simulink model "MDCC"  (R2021b)
settings: Solver=FixedStepDiscrete  StartTime=0.0  StopTime=10.0  FixedStep=0.0001  RelTol=1e-3
model workspace (MATLAB code in the model file):
  | cmdLim = Simulink.Parameter;
  | cmdLim.Value = 15;
  | cmdLim.Description = 'Limit for controlling the maximum surface command angle.';
  | cmdLim.Min = 0;
  | cmdLim.Max = 90;
  | cmdLim.DocUnits = 'deg';
  | 
  | dispGain = Simulink.Parameter;
  | dispGain.Value = 0.75;
  | dispGain.Description = 'Gain applied to the displacement error.';
  | dispGain.Min = 0;
  | dispGain.Max = [];
  | dispGain.DocUnits = 'deg/sec/deg';
  | 
  | dispLim = Simulink.Parameter;
  | dispLim.Value = 30;
  | dispLim.Description = 'Limit for controlling the maximum commanded angle.';
  | dispLim.Min = 0;
  | dispLim.Max = 180;
  | dispLim.DocUnits = 'deg';
  | 
  | intGain = Simulink.Parameter;
  | intGain.Value = 0.5;
  | intGain.Description = 'Gain applied to the integral error.';
  | intGain.Min = 0;
  | intGain.Max = [];
  | intGain.DocUnits = 'deg/sec/deg/sec';
  | 
  | intLim = Simulink.Parameter;
  | intLim.Value = 5;
  | intLim.Description = 'Limit for controlling the maximum commanded angle.';
  | intLim.Min = 0;
  | intLim.Max = 90;
  | intLim.DocUnits = 'deg';
  | 
  | rateGain = Simulink.Parameter;
  | rateGain.Value = 2;
  | rateGain.Description = 'Gain applied to the rate error.';
  | rateGain.Min = 0;
  | rateGain.Max = [];
  | rateGain.DocUnits = 'deg/deg/sec';
  | 
  | rateLim = Simulink.Parameter;
  | rateLim.Value = 6;
  | rateLim.Description = 'Limit for controlling the maximum commanded angle.';
  | rateLim.Min = 0;
  | rateLim.Max = 180;
  | rateLim.DocUnits = 'deg/sec';
  | 
  | hdgGain = Simulink.Parameter;
  | hdgGain.Value = 0.015;
values from neighbouring files (symbols this model uses):
  KfDeadCompen_SetDeltaTime_us = myPackage.Parameter    [DeadCompen.m]
  Ts = 5E-6    (= 5e-06)    [iPMSM_data.m]
  VbDeadComp_SwtUseIsttrDes_flg = myPackage.Parameter    [DeadCompen.m]
  VfDeadCompen_ISttrDdeThdSwt_A = myPackage.Parameter    [DeadCompen.m]
  VfDeadCompen_ISttrIgbtThdSwt_A = myPackage.Parameter    [DeadCompen.m]
  VfDeadCompen_rDdeISttrHi_R = myPackage.Parameter    [DeadCompen.m]
  VfDeadCompen_rDdeISttrLo_R = myPackage.Parameter    [DeadCompen.m]
  VfDeadCompen_rIgbtISttrHi_R = myPackage.Parameter    [DeadCompen.m]
  VfDeadCompen_rIgbtISttrLo_R = myPackage.Parameter    [DeadCompen.m]
  VfDeadCompen_uDdeISttrHi_V = myPackage.Parameter    [DeadCompen.m]
  VfDeadCompen_uDdeISttrLo_V = myPackage.Parameter    [DeadCompen.m]
  VfDeadCompen_uIgbtISttrHi_V = myPackage.Parameter    [DeadCompen.m]
  VfDeadCompen_uIgbtISttrLo_V = myPackage.Parameter    [DeadCompen.m]
undefined symbols (not defined in the file or in its folder): CosTable12bit_Y, GLBCal_GLBCal_Kf_DCLinkOverVolErrThd_V, GLBCal_GLBCal_Kf_DCLinkUnderVolErrThd_V, GLBCal_GLBCal_Kf_EquiLd_NULL, GLBCal_GLBCal_Kf_EquiLq_NULL, GLBCal_GLBCal_Kf_MotorRatedSpeed_rpm, GLBCal_GLBCal_Kf_MotorSpeedHysteresis_Coef, GLBCal_Ke_MotorPolePairsNum_NULL, IoHwAbOpArg_PwmDutyCyclePhU_NULL, IoHwAbOpArg_PwmDutyCyclePhV_NULL, IoHwAbOpArg_PwmDutyCyclePhW_NULL, IoHwAbOpArg_PwmOutputEn, KbMDCC_DeadTimeCompEn_flg, KbMDCC_MCF_flgHarmInIsdqTab11ZR_flg, KbMDCC_MCF_flgHarmInIsdqTab13ZR_flg, KbMDCC_MCF_flgHarmInIsdqTab5ZR_flg, KbMDCC_MCF_flgHarmInIsdqTab7ZR_flg, KbMDCC_MCF_flgHarmInject_flg, KbMDCC_SetEAngleEn_flg, KbMDCC_UdUqFwOmit_flg, KfDeadCompen_CpPeriodTimesT_NULL, KfMDCC_ActiveDischargeIdCurVal_A, KfMDCC_ActiveDischargeIqCurVal_A, KfMDCC_DCLinkVolRate_coef, KfMDCC_DebugEAngleInit_rad, KfMDCC_DebugUalphaVolCmd_V, KfMDCC_DebugUbetaVolCmd_V, KfMDCC_DebugUdCmd_V, KfMDCC_DebugUqCmd_V, KfMDCC_DebugUsCmd_V, KfMDCC_DebugUsRate_V, KfMDCC_IMCResp_NULL, KfMDCC_IMCStab_NULL, KfMDCC_InvParkCpPeriodTimesT_NULL, KfMDCC_MCF_CircAge_NULL, KfMDCC_MCF_flgUse11Harm_flg, KfMDCC_MCF_flgUse13Harm_flg, KfMDCC_MCF_flgUse5Harm_flg, KfMDCC_MCF_flgUse7Harm_flg, KfMDCC_MCF_Harm1113FLParamSpeedThrd_rads, KfMDCC_MCF_Harm57FLParamSpeedThrd_rads, KfMDCC_MCF_HarmcofFltN_NULL, KfMDCC_MCF_HarmCpnAg_NULL, KfMDCC_MCF_HarmfLParaHigh_coef, KfMDCC_MCF_HarmfLParaLow_coef, KfMDCC_MCF_HarmIn1113ZRY_Trq_Nm, KfMDCC_MCF_HarmIn11_SpdLimHigh_rads, KfMDCC_MCF_HarmIn11_SpdLimLow_rads, KfMDCC_MCF_HarmIn11ZRY_Isd_A, KfMDCC_MCF_HarmIn11ZRY_Isq_A, KfMDCC_MCF_HarmIn13_SpdLimHigh_rads, KfMDCC_MCF_HarmIn13_SpdLimLow_rads, KfMDCC_MCF_HarmIn13ZRY_Isd_A, KfMDCC_MCF_HarmIn13ZRY_Isq_A, KfMDCC_MCF_HarmIn57ZRY_Trq_Nm, KfMDCC_MCF_HarmIn5_SpdLimHigh_rads, KfMDCC_MCF_HarmIn5_SpdLimLow_rads, KfMDCC_MCF_HarmIn5ZRY_Isd_A, KfMDCC_MCF_HarmIn5ZRY_Isq_A, KfMDCC_MCF_HarmIn7_SpdLimHigh_rads ... (+47)
libraries: simulink x40, PMSM_Library x3, mcbcontrolslib x1
(part 5 of 8)

== system MDCC/DoCurCtr_sys/MDCC/UdUqCalc_Sys/MDCC_MCF_Sys/Enabled Subsystem/Harmonic_Injection_11/Subsystem ==
  MCF_Harm_isdDes11 : Inport
  MCF_Harm_isqDes11 : Inport  Port=2
  MCF_Harm_isdAct11 : Inport  Port=3
  MCF_Harm_isqAct11 : Inport  Port=4
  MCF_Sin11Ag : Inport  Port=5
  MCF_Cos11Ag : Inport  Port=6
  Rdc_absnWoFlt_rads : Inport  Port=7
  MCF_flgHarm11PIRest : Inport  Port=8
  ZeroEnable : EnablePort
  Harm_11Step_KpKi : Subsystem
  RevPark : Subsystem
  MCF_uAlpha_Harm11 : Outport  VectorParamsAs1DForOutWhenUnconnected=off
  MCF_uBeta_Harm11 : Outport  Port=2  VectorParamsAs1DForOutWhenUnconnected=off
  wires:
  MCF_Harm_isqDes11/1 -> Harm_11Step_KpKi/2(MCF_Harm_isqDes11)
  MCF_Harm_isqAct11/1 -> Harm_11Step_KpKi/4(MCF_Harm_isqAct11)
  RevPark/2(MCF_uBeta_Harm11) -> MCF_uBeta_Harm11/1
  MCF_Harm_isdAct11/1 -> Harm_11Step_KpKi/3(MCF_Harm_isdAct11)
  RevPark/1(MCF_uAlpha_Harm11) -> MCF_uAlpha_Harm11/1
  MCF_Harm_isdDes11/1 -> Harm_11Step_KpKi/1(MCF_Harm_isdDes11)
  MCF_flgHarm11PIRest/1 -> Harm_11Step_KpKi/6(MCF_flgHarm11PIRest)
  Rdc_absnWoFlt_rads/1 -> Harm_11Step_KpKi/5(Rdc_absnWoFlt_rads)
  Harm_11Step_KpKi/1(MCF_Harm_ud11PI) -> RevPark/1(MCF_Harm_ud11PI)
  Harm_11Step_KpKi/2(MCF_Harm_uq11PI) -> RevPark/2(MCF_Harm_uq11PI)
  MCF_Sin11Ag/1 -> RevPark/3(MCF_Sin11Ag)
  MCF_Cos11Ag/1 -> RevPark/4(MCF_Cos11Ag)

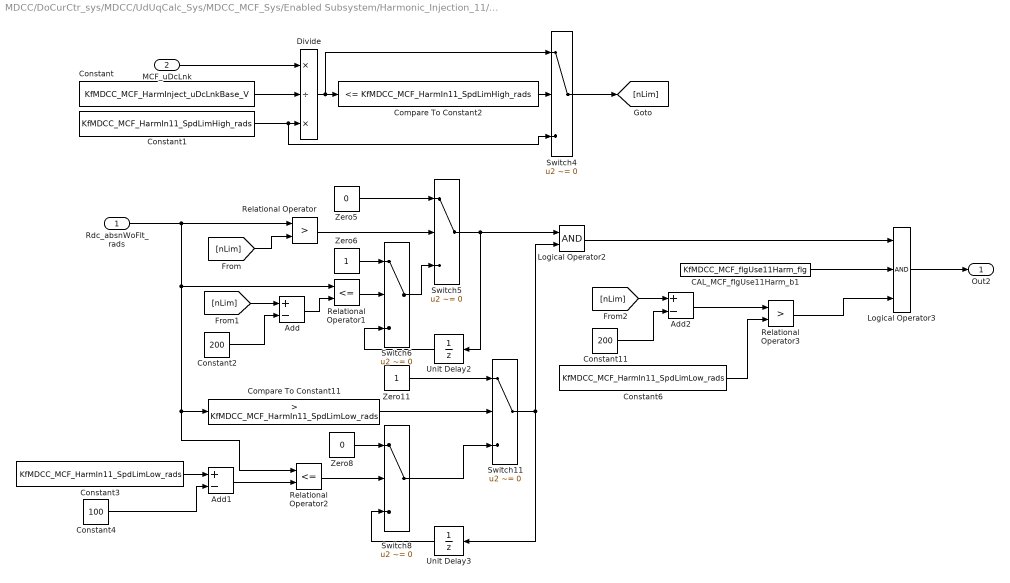
== system MDCC/DoCurCtr_sys/MDCC/UdUqCalc_Sys/MDCC_MCF_Sys/Enabled Subsystem/Harmonic_Injection_11/Subsystem1 ==
  Rdc_absnWoFlt_rads : Inport
  MCF_uDcLnk : Inport  Port=2
  Add : Sum  Inputs=+-
  Add1 : Sum  Inputs=+-
  Add2 : Sum  Inputs=+-
  CAL_MCF_flgUse11Harm_b1 : Constant  Value=KfMDCC_MCF_flgUse11Harm_flg
  Compare To Constant11 : simulink/Logic and Bit Operations/Compare To Constant  relop=>  const=KfMDCC_MCF_HarmIn11_SpdLimLow_rads  OutDataTypeStr=boolean
  Compare To Constant2 : simulink/Logic and Bit Operations/Compare To Constant  relop=<=  const=KfMDCC_MCF_HarmIn11_SpdLimHigh_rads  OutDataTypeStr=boolean
  Constant : Constant  Value=KfMDCC_MCF_HarmInject_uDcLnkBase_V
  Constant1 : Constant  Value=KfMDCC_MCF_HarmIn11_SpdLimHigh_rads
  Constant11 : Constant  Value=200  OutDataTypeStr=single
  Constant2 : Constant  Value=200  OutDataTypeStr=single
  Constant3 : Constant  Value=KfMDCC_MCF_HarmIn11_SpdLimLow_rads
  Constant4 : Constant  Value=100  OutDataTypeStr=single
  Constant6 : Constant  Value=KfMDCC_MCF_HarmIn11_SpdLimLow_rads
  Divide : Product  Inputs=*/*
  Logical Operator2 : Logic  AllPortsSameDT=off  OutDataTypeStr=boolean
  Logical Operator3 : Logic  Inputs=3  AllPortsSameDT=off  OutDataTypeStr=boolean
  Relational Operator : RelationalOperator  Operator=>  OutDataTypeStr=boolean  RndMeth=Simplest
  Relational Operator1 : RelationalOperator  Operator=<=  OutDataTypeStr=boolean  RndMeth=Simplest
  Relational Operator2 : RelationalOperator  Operator=<=  OutDataTypeStr=boolean  RndMeth=Simplest
  Relational Operator3 : RelationalOperator  Operator=>  OutDataTypeStr=boolean  RndMeth=Simplest
  Switch{4..6,8,11} (5 alike) : Switch  Criteria=u2 ~= 0
  Unit Delay2 : UnitDelay  SampleTime=-1  HasFrameUpgradeWarning=on
  Unit Delay3 : UnitDelay  SampleTime=-1  HasFrameUpgradeWarning=on
  Zero11 : Constant  OutDataTypeStr=boolean
  Zero5 : Constant  Value=0  OutDataTypeStr=boolean
  Zero6 : Constant  OutDataTypeStr=boolean
  Zero8 : Constant  Value=0  OutDataTypeStr=boolean
  Out2 : Outport
  wires:
  Constant/1 -> Divide/2
  MCF_uDcLnk/1 -> Divide/1
  Constant1/1 -> Switch4/3, Divide/3
  Divide/1 -> Switch4/1, Compare To Constant2/1
  Compare To Constant2/1 -> Switch4/2
  Switch4/1 -> [nLim]
  CAL_MCF_flgUse11Harm_b1/1 -> Logical Operator3/2
  Relational Operator2/1 -> Switch8/2
  Relational Operator1/1 -> Switch6/2
  Switch8/1 -> Switch11/3
  Compare To Constant11/1 -> Switch11/2
  Unit Delay3/1 -> Switch8/3
  Switch11/1 -> Unit Delay3/1, Logical Operator2/2
  Relational Operator/1 -> Switch5/2
  Switch5/1 -> Logical Operator2/1, Unit Delay2/1
  Zero6/1 -> Switch6/1
  Logical Operator3/1 -> Out2/1
  Switch6/1 -> Switch5/3
  Zero11/1 -> Switch11/1
  Unit Delay2/1 -> Switch6/3
  Zero8/1 -> Switch8/1
  Rdc_absnWoFlt_rads/1 -> Relational Operator/1, Relational Operator2/1, Compare To Constant11/1, Relational Operator1/1
  Logical Operator2/1 -> Logical Operator3/1
  Zero5/1 -> Switch5/1
  [nLim] -> Relational Operator/2
  [nLim] -> Add/1
  Add/1 -> Relational Operator1/2
  Constant2/1 -> Add/2
  Constant3/1 -> Add1/1
  Constant4/1 -> Add1/2
  Add1/1 -> Relational Operator2/2
  [nLim] -> Add2/1
  Constant11/1 -> Add2/2
  Add2/1 -> Relational Operator3/1
  Constant6/1 -> Relational Operator3/2
  Relational Operator3/1 -> Logical Operator3/3

== system MDCC/DoCurCtr_sys/MDCC/UdUqCalc_Sys/MDCC_MCF_Sys/Enabled Subsystem/Harmonic_Injection_11/Subsystem2 ==
  TDC_TrqDes : Inport
  flgHarmUse : Inport  Port=2
  Add : Sum  Inputs=+-
  Add1 : Sum  Inputs=-+
  Add2 : Sum  Inputs=-+
  Add3 : Sum
  Compare To Constant : simulink/Logic and Bit Operations/Compare To Constant  relop=>=  const=KfMDCC_MCF_TrqFltCof_NULL  OutDataTypeStr=boolean
  Compare To Constant1 : simulink/Logic and Bit Operations/Compare To Constant  relop=>=  const=KfMDCC_MCF_TrqFltCof_NULL  OutDataTypeStr=boolean
  Constant : Constant  Value=KfMDCC_MCF_TrqFlt_coef  OutDataTypeStr=single
  Switch : Switch  Criteria=u2 > Threshold
  Switch1 : Switch  Criteria=u2 > Threshold
  Switch2 : Switch  Criteria=u2 ~= 0
  Unit Delay : UnitDelay  SampleTime=-1  HasFrameUpgradeWarning=on
  Unit Delay1 : UnitDelay  SampleTime=-1  HasFrameUpgradeWarning=on
  Zero : Constant  Value=0  OutDataTypeStr=single
  TDC_TrqDesFlt : Outport
  wires:
  Add/1 -> Compare To Constant/1
  Compare To Constant/1 -> Switch/2
  Add1/1 -> Switch/1
  Switch/1 -> Switch2/1
  TDC_TrqDes/1 -> Switch1/3, Add2/2, Add/2
  Add2/1 -> Compare To Constant1/1
  Constant/1 -> Add1/1, Add3/1
  Add3/1 -> Switch1/1
  Compare To Constant1/1 -> Switch1/2
  Switch1/1 -> Switch/3
  Unit Delay/1 -> Add/1, Add1/2, Add2/1, Add3/2
  flgHarmUse/1 -> Unit Delay1/1
  Unit Delay1/1 -> Switch2/2
  Zero/1 -> Switch2/3
  Switch2/1 -> Unit Delay/1, TDC_TrqDesFlt/1

== system MDCC/DoCurCtr_sys/MDCC/UdUqCalc_Sys/MDCC_MCF_Sys/Enabled Subsystem/Harmonic_Injection_13/Set_13_steps_current_isdqdes ==
  TDC_TrqDesFlt : Inport
  1-D Lookup Table : Lookup_n-D  NumberOfTableDimensions=1  BreakpointsForDimension1=KfMDCC_MCF_HarmIn1113ZRY_Trq_Nm  Table=KfMDCC_MCF_HarmIn13ZRY_Isd_A  InternalRulePriority=Speed  RndMeth=Simplest  InputSameDT=on
  1-D Lookup Table1 : Lookup_n-D  NumberOfTableDimensions=1  BreakpointsForDimension1=KfMDCC_MCF_HarmIn1113ZRY_Trq_Nm  Table=KfMDCC_MCF_HarmIn13ZRY_Isq_A  InternalRulePriority=Speed  RndMeth=Simplest  InputSameDT=on
  Bus Creator1 : BusCreator  Inputs=2
  Bus Creator2 : BusCreator  Inputs=2
  Bus Selector1 : BusSelector  OutputSignals=MCF_IsdDes13Harm_A,MCF_IsqDes13Harm_A
  CAL_MCF_IsDes13Harm_f32 : Constant  Value=KfMDCC_MCF_IsDes13Harm_A
  CAL_MCF_IsThetaDes13Harm_f32 : Constant  Value=KfMDCC_MCF_IsThetaDes13Harm_NULL
  CAL_MCF_flgHarmInIsdqTab13ZR_b : Constant  Value=KbMDCC_MCF_flgHarmInIsdqTab13ZR_flg
  LookUpEAngleCosSin2 : Subsystem  TreatAsAtomicUnit=on  RTWFcnName=MCF_MDCC_LookUpEAngleCosSin  RTWFileName=MDCC
      settings: RTWFcnNameOpts=User specified
  Product13 : Product  OutDataTypeStr=uint16
  Product2 : Product
  Product5 : Product
  Signal Copy : SignalConversion  OverrideOpt=off
  Signal Copy1 : SignalConversion  OverrideOpt=off
  Sine_and_cosine_table1 : Constant  Value=13.31313  OutDataTypeStr=single
  Switch1 : Switch  Criteria=u2 ~= 0
  VfMDCC_MCF_IsdDes13Harm_A : Outport  VectorParamsAs1DForOutWhenUnconnected=off
  VfMDCC_MCF_IsqDes13Harm_A : Outport  Port=2  VectorParamsAs1DForOutWhenUnconnected=off
  wires:
  Signal Copy1/1 -> VfMDCC_MCF_IsqDes13Harm_A/1  "VfMDCC_MCF_IsqDes13Harm_A"
  Signal Copy/1 -> VfMDCC_MCF_IsdDes13Harm_A/1  "VfMDCC_MCF_IsdDes13Harm_A"
  Bus Selector1/2 -> Signal Copy1/1  "<MCF_IsqDes13Harm_A>"
  Bus Selector1/1 -> Signal Copy/1  "<MCF_IsdDes13Harm_A>"
  Switch1/1 -> Bus Selector1/1
  CAL_MCF_flgHarmInIsdqTab13ZR_b/1 -> Switch1/2
  1-D Lookup Table1/1 -> Bus Creator2/2  "MCF_IsqDes13Harm_A"
  Bus Creator2/1 -> Switch1/1
  1-D Lookup Table/1 -> Bus Creator2/1  "MCF_IsdDes13Harm_A"
  TDC_TrqDesFlt/1 -> 1-D Lookup Table/1, 1-D Lookup Table1/1
  CAL_MCF_IsDes13Harm_f32/1 -> Product5/1, Product2/1
  Sine_and_cosine_table1/1 -> Product13/2
  LookUpEAngleCosSin2/2(VfMDCC_EAngleSin_NULL) -> Product5/2
  Product2/1 -> Bus Creator1/1  "MCF_IsdDes13Harm_A"
  Bus Creator1/1 -> Switch1/3
  Product13/1 -> LookUpEAngleCosSin2/1(VuMDCC_MotorPositionCnt_NULL)
  CAL_MCF_IsThetaDes13Harm_f32/1 -> Product13/1
  Product5/1 -> Bus Creator1/2  "MCF_IsqDes13Harm_A"
  LookUpEAngleCosSin2/1(VfMDCC_EAngleCos_NULL) -> Product2/2

== system MDCC/DoCurCtr_sys/MDCC/UdUqCalc_Sys/MDCC_MCF_Sys/Enabled Subsystem/Harmonic_Injection_13/Subsystem ==
  MCF_Harm_isdDes13 : Inport
  MCF_Harm_isqDes13 : Inport  Port=2
  MCF_Harm_isdAct13 : Inport  Port=3
  MCF_Harm_isqAct13 : Inport  Port=4
  MCF_Sin13Ag : Inport  Port=5
  MCF_Cos13Ag : Inport  Port=6
  Rdc_absnWoFlt_rads : Inport  Port=7
  MCF_flgHarm13PIRest : Inport  Port=8
  ZeroEnable : EnablePort
  Harm_13Step_KpKi : Subsystem
  RevPark : Subsystem
  MCF_uAlpha_Harm13 : Outport  VectorParamsAs1DForOutWhenUnconnected=off
  MCF_uBeta_Harm13 : Outport  Port=2  VectorParamsAs1DForOutWhenUnconnected=off
  wires:
  MCF_Harm_isqDes13/1 -> Harm_13Step_KpKi/2(MCF_Harm_isqDes13)
  MCF_Harm_isqAct13/1 -> Harm_13Step_KpKi/4(MCF_Harm_isqAct13)
  RevPark/2(MCF_uBeta_Harm13) -> MCF_uBeta_Harm13/1
  MCF_Harm_isdAct13/1 -> Harm_13Step_KpKi/3(MCF_Harm_isdAct13)
  RevPark/1(MCF_uAlpha_Harm13) -> MCF_uAlpha_Harm13/1
  MCF_Harm_isdDes13/1 -> Harm_13Step_KpKi/1(MCF_Harm_isdDes13)
  MCF_flgHarm13PIRest/1 -> Harm_13Step_KpKi/6(MCF_flgHarm13PIRest)
  Rdc_absnWoFlt_rads/1 -> Harm_13Step_KpKi/5(Rdc_absnWoFlt_rads)
  Harm_13Step_KpKi/1(MCF_Harm_ud13PI) -> RevPark/1(MCF_Harm_ud13PI)
  Harm_13Step_KpKi/2(MCF_Harm_uq13PI) -> RevPark/2(MCF_Harm_uq13PI)
  MCF_Sin13Ag/1 -> RevPark/3(MCF_Sin13Ag)
  MCF_Cos13Ag/1 -> RevPark/4(MCF_Cos13Ag)

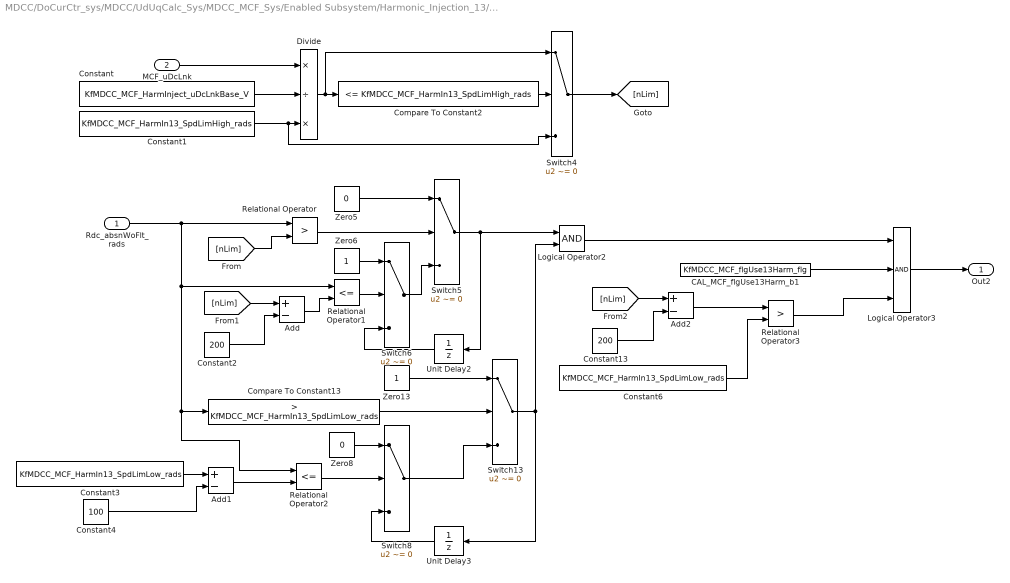
== system MDCC/DoCurCtr_sys/MDCC/UdUqCalc_Sys/MDCC_MCF_Sys/Enabled Subsystem/Harmonic_Injection_13/Subsystem1 ==
  Rdc_absnWoFlt_rads : Inport
  MCF_uDcLnk : Inport  Port=2
  Add : Sum  Inputs=+-
  Add1 : Sum  Inputs=+-
  Add2 : Sum  Inputs=+-
  CAL_MCF_flgUse13Harm_b1 : Constant  Value=KfMDCC_MCF_flgUse13Harm_flg
  Compare To Constant13 : simulink/Logic and Bit Operations/Compare To Constant  relop=>  const=KfMDCC_MCF_HarmIn13_SpdLimLow_rads  OutDataTypeStr=boolean
  Compare To Constant2 : simulink/Logic and Bit Operations/Compare To Constant  relop=<=  const=KfMDCC_MCF_HarmIn13_SpdLimHigh_rads  OutDataTypeStr=boolean
  Constant : Constant  Value=KfMDCC_MCF_HarmInject_uDcLnkBase_V
  Constant1 : Constant  Value=KfMDCC_MCF_HarmIn13_SpdLimHigh_rads
  Constant13 : Constant  Value=200  OutDataTypeStr=single
  Constant2 : Constant  Value=200  OutDataTypeStr=single
  Constant3 : Constant  Value=KfMDCC_MCF_HarmIn13_SpdLimLow_rads
  Constant4 : Constant  Value=100  OutDataTypeStr=single
  Constant6 : Constant  Value=KfMDCC_MCF_HarmIn13_SpdLimLow_rads
  Divide : Product  Inputs=*/*
  Logical Operator2 : Logic  AllPortsSameDT=off  OutDataTypeStr=boolean
  Logical Operator3 : Logic  Inputs=3  AllPortsSameDT=off  OutDataTypeStr=boolean
  Relational Operator : RelationalOperator  Operator=>  OutDataTypeStr=boolean  RndMeth=Simplest
  Relational Operator1 : RelationalOperator  Operator=<=  OutDataTypeStr=boolean  RndMeth=Simplest
  Relational Operator2 : RelationalOperator  Operator=<=  OutDataTypeStr=boolean  RndMeth=Simplest
  Relational Operator3 : RelationalOperator  Operator=>  OutDataTypeStr=boolean  RndMeth=Simplest
  Switch{4..6,8,13} (5 alike) : Switch  Criteria=u2 ~= 0
  Unit Delay2 : UnitDelay  SampleTime=-1  HasFrameUpgradeWarning=on
  Unit Delay3 : UnitDelay  SampleTime=-1  HasFrameUpgradeWarning=on
  Zero13 : Constant  OutDataTypeStr=boolean
  Zero5 : Constant  Value=0  OutDataTypeStr=boolean
  Zero6 : Constant  OutDataTypeStr=boolean
  Zero8 : Constant  Value=0  OutDataTypeStr=boolean
  Out2 : Outport
  wires:
  Constant/1 -> Divide/2
  MCF_uDcLnk/1 -> Divide/1
  Constant1/1 -> Switch4/3, Divide/3
  Divide/1 -> Switch4/1, Compare To Constant2/1
  Compare To Constant2/1 -> Switch4/2
  Switch4/1 -> [nLim]
  CAL_MCF_flgUse13Harm_b1/1 -> Logical Operator3/2
  Relational Operator2/1 -> Switch8/2
  Relational Operator1/1 -> Switch6/2
  Switch8/1 -> Switch13/3
  Compare To Constant13/1 -> Switch13/2
  Unit Delay3/1 -> Switch8/3
  Switch13/1 -> Unit Delay3/1, Logical Operator2/2
  Relational Operator/1 -> Switch5/2
  Switch5/1 -> Logical Operator2/1, Unit Delay2/1
  Zero6/1 -> Switch6/1
  Logical Operator3/1 -> Out2/1
  Switch6/1 -> Switch5/3
  Zero13/1 -> Switch13/1
  Unit Delay2/1 -> Switch6/3
  Zero8/1 -> Switch8/1
  Rdc_absnWoFlt_rads/1 -> Relational Operator/1, Relational Operator2/1, Compare To Constant13/1, Relational Operator1/1
  Logical Operator2/1 -> Logical Operator3/1
  Zero5/1 -> Switch5/1
  [nLim] -> Relational Operator/2
  [nLim] -> Add/1
  Add/1 -> Relational Operator1/2
  Constant2/1 -> Add/2
  Constant3/1 -> Add1/1
  Constant4/1 -> Add1/2
  Add1/1 -> Relational Operator2/2
  [nLim] -> Add2/1
  Constant13/1 -> Add2/2
  Add2/1 -> Relational Operator3/1
  Constant6/1 -> Relational Operator3/2
  Relational Operator3/1 -> Logical Operator3/3

== system MDCC/DoCurCtr_sys/MDCC/UdUqCalc_Sys/MDCC_MCF_Sys/Enabled Subsystem/Harmonic_Injection_13/Subsystem2 ==
  TDC_TrqDes : Inport
  flgHarmUse : Inport  Port=2
  Add : Sum  Inputs=+-
  Add1 : Sum  Inputs=-+
  Add2 : Sum  Inputs=-+
  Add3 : Sum
  Compare To Constant : simulink/Logic and Bit Operations/Compare To Constant  relop=>=  const=KfMDCC_MCF_TrqFltCof_NULL  OutDataTypeStr=boolean
  Compare To Constant1 : simulink/Logic and Bit Operations/Compare To Constant  relop=>=  const=KfMDCC_MCF_TrqFltCof_NULL  OutDataTypeStr=boolean
  Constant : Constant  Value=KfMDCC_MCF_TrqFlt_coef  OutDataTypeStr=single
  Switch : Switch  Criteria=u2 > Threshold
  Switch1 : Switch  Criteria=u2 > Threshold
  Switch2 : Switch  Criteria=u2 ~= 0
  Unit Delay : UnitDelay  SampleTime=-1  HasFrameUpgradeWarning=on
  Unit Delay1 : UnitDelay  SampleTime=-1  HasFrameUpgradeWarning=on
  Zero : Constant  Value=0  OutDataTypeStr=single
  TDC_TrqDesFlt : Outport
  wires:
  Add/1 -> Compare To Constant/1
  Compare To Constant/1 -> Switch/2
  Add1/1 -> Switch/1
  Switch/1 -> Switch2/1
  TDC_TrqDes/1 -> Switch1/3, Add2/2, Add/2
  Add2/1 -> Compare To Constant1/1
  Constant/1 -> Add1/1, Add3/1
  Add3/1 -> Switch1/1
  Compare To Constant1/1 -> Switch1/2
  Switch1/1 -> Switch/3
  Unit Delay/1 -> Add/1, Add1/2, Add2/1, Add3/2
  flgHarmUse/1 -> Unit Delay1/1
  Unit Delay1/1 -> Switch2/2
  Zero/1 -> Switch2/3
  Switch2/1 -> Unit Delay/1, TDC_TrqDesFlt/1

== system MDCC/DoCurCtr_sys/MDCC/UdUqCalc_Sys/MDCC_MCF_Sys/Enabled Subsystem/Harmonic_Injection_5/Set_5_steps_current_isdqdes ==
  TDC_TrqDesFlt : Inport
  1-D Lookup Table : Lookup_n-D  NumberOfTableDimensions=1  BreakpointsForDimension1=KfMDCC_MCF_HarmIn57ZRY_Trq_Nm  Table=KfMDCC_MCF_HarmIn5ZRY_Isd_A  InternalRulePriority=Speed  RndMeth=Simplest  InputSameDT=on
  1-D Lookup Table1 : Lookup_n-D  NumberOfTableDimensions=1  BreakpointsForDimension1=KfMDCC_MCF_HarmIn57ZRY_Trq_Nm  Table=KfMDCC_MCF_HarmIn5ZRY_Isq_A  InternalRulePriority=Speed  RndMeth=Simplest  InputSameDT=on
  Bus Creator1 : BusCreator  Inputs=2
  Bus Creator2 : BusCreator  Inputs=2
  Bus Selector1 : BusSelector  OutputSignals=MCF_IsdDes5Harm_A,MCF_IsqDes5Harm_A
  CAL_MCF_IsDes5Harm_f32 : Constant  Value=KfMDCC_MCF_IsDes5Harm_A
  CAL_MCF_IsThetaDes5Harm_f32 : Constant  Value=KfMDCC_MCF_IsThetaDes5Harm_NULL
  CAL_MCF_flgHarmInIsdqTab5ZR_b : Constant  Value=KbMDCC_MCF_flgHarmInIsdqTab5ZR_flg
  LookUpEAngleCosSin2 : Subsystem  TreatAsAtomicUnit=on  RTWFcnName=MCF_MDCC_LookUpEAngleCosSin  RTWFileName=MDCC
      settings: RTWFcnNameOpts=User specified
  Product2 : Product
  Product5 : Product
  Product7 : Product  OutDataTypeStr=uint16
  Signal Copy : SignalConversion  OverrideOpt=off
  Signal Copy1 : SignalConversion  OverrideOpt=off
  Sine_and_cosine_table1 : Constant  Value=11.375  OutDataTypeStr=single
  Switch1 : Switch  Criteria=u2 ~= 0
  VfMDCC_MCF_IsdDes5Harm_A : Outport  VectorParamsAs1DForOutWhenUnconnected=off
  VfMDCC_MCF_IsqDes5Harm_A : Outport  Port=2  VectorParamsAs1DForOutWhenUnconnected=off
  wires:
  Signal Copy1/1 -> VfMDCC_MCF_IsqDes5Harm_A/1  "VfMDCC_MCF_IsqDes5Harm_A"
  Signal Copy/1 -> VfMDCC_MCF_IsdDes5Harm_A/1  "VfMDCC_MCF_IsdDes5Harm_A"
  Bus Selector1/2 -> Signal Copy1/1  "<MCF_IsqDes5Harm_A>"
  Bus Selector1/1 -> Signal Copy/1  "<MCF_IsdDes5Harm_A>"
  Switch1/1 -> Bus Selector1/1
  CAL_MCF_flgHarmInIsdqTab5ZR_b/1 -> Switch1/2
  1-D Lookup Table1/1 -> Bus Creator2/2  "MCF_IsqDes5Harm_A"
  Bus Creator2/1 -> Switch1/1
  1-D Lookup Table/1 -> Bus Creator2/1  "MCF_IsdDes5Harm_A"
  TDC_TrqDesFlt/1 -> 1-D Lookup Table/1, 1-D Lookup Table1/1
  CAL_MCF_IsDes5Harm_f32/1 -> Product5/1, Product2/1
  Sine_and_cosine_table1/1 -> Product7/2
  LookUpEAngleCosSin2/2(VfMDCC_EAngleSin_NULL) -> Product5/2
  Product2/1 -> Bus Creator1/1  "MCF_IsdDes5Harm_A"
  Bus Creator1/1 -> Switch1/3
  Product7/1 -> LookUpEAngleCosSin2/1(VuMDCC_MotorPositionCnt_NULL)
  CAL_MCF_IsThetaDes5Harm_f32/1 -> Product7/1
  Product5/1 -> Bus Creator1/2  "MCF_IsqDes5Harm_A"
  LookUpEAngleCosSin2/1(VfMDCC_EAngleCos_NULL) -> Product2/2

== system MDCC/DoCurCtr_sys/MDCC/UdUqCalc_Sys/MDCC_MCF_Sys/Enabled Subsystem/Harmonic_Injection_5/Subsystem ==
  MCF_Harm_isdDes5 : Inport
  MCF_Harm_isqDes5 : Inport  Port=2
  MCF_Harm_isdAct5 : Inport  Port=3
  MCF_Harm_isqAct5 : Inport  Port=4
  MCF_Sin5Ag : Inport  Port=5
  MCF_Cos5Ag : Inport  Port=6
  Rdc_absnWoFlt_rads : Inport  Port=7
  MCF_flgHarm5PIRest : Inport  Port=8
  ZeroEnable : EnablePort
  Harm_5Step_KpKi : Subsystem
  RevPark : Subsystem
  MCF_uAlpha_Harm5 : Outport  VectorParamsAs1DForOutWhenUnconnected=off
  MCF_uBeta_Harm5 : Outport  Port=2  VectorParamsAs1DForOutWhenUnconnected=off
  wires:
  MCF_Harm_isqDes5/1 -> Harm_5Step_KpKi/2(MCF_Harm_isqDes5)
  MCF_Harm_isqAct5/1 -> Harm_5Step_KpKi/4(MCF_Harm_isqAct5)
  RevPark/2(MCF_uBeta_Harm5) -> MCF_uBeta_Harm5/1
  MCF_Harm_isdAct5/1 -> Harm_5Step_KpKi/3(MCF_Harm_isdAct5)
  RevPark/1(MCF_uAlpha_Harm5) -> MCF_uAlpha_Harm5/1
  MCF_Harm_isdDes5/1 -> Harm_5Step_KpKi/1(MCF_Harm_isdDes5)
  MCF_flgHarm5PIRest/1 -> Harm_5Step_KpKi/6(MCF_flgHarm5PIRest)
  Rdc_absnWoFlt_rads/1 -> Harm_5Step_KpKi/5(Rdc_absnWoFlt_rads)
  Harm_5Step_KpKi/1(MCF_Harm_ud5PI) -> RevPark/1(MCF_Harm_ud5PI)
  Harm_5Step_KpKi/2(MCF_Harm_uq5PI) -> RevPark/2(MCF_Harm_uq5PI)
  MCF_Sin5Ag/1 -> RevPark/3(MCF_Sin5Ag)
  MCF_Cos5Ag/1 -> RevPark/4(MCF_Cos5Ag)

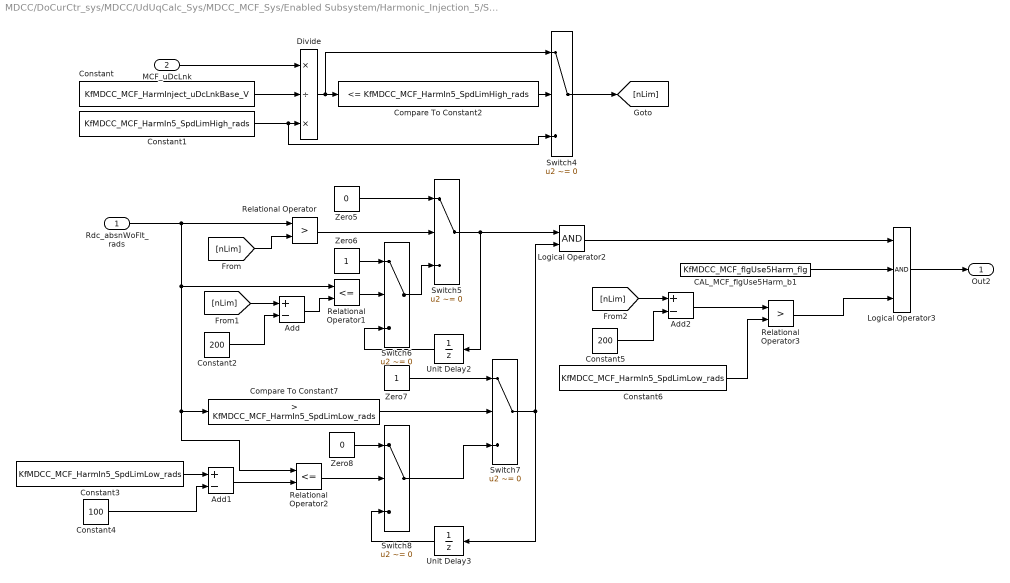
== system MDCC/DoCurCtr_sys/MDCC/UdUqCalc_Sys/MDCC_MCF_Sys/Enabled Subsystem/Harmonic_Injection_5/Subsystem1 ==
  Rdc_absnWoFlt_rads : Inport
  MCF_uDcLnk : Inport  Port=2
  Add : Sum  Inputs=+-
  Add1 : Sum  Inputs=+-
  Add2 : Sum  Inputs=+-
  CAL_MCF_flgUse5Harm_b1 : Constant  Value=KfMDCC_MCF_flgUse5Harm_flg
  Compare To Constant2 : simulink/Logic and Bit Operations/Compare To Constant  relop=<=  const=KfMDCC_MCF_HarmIn5_SpdLimHigh_rads  OutDataTypeStr=boolean
  Compare To Constant7 : simulink/Logic and Bit Operations/Compare To Constant  relop=>  const=KfMDCC_MCF_HarmIn5_SpdLimLow_rads  OutDataTypeStr=boolean
  Constant : Constant  Value=KfMDCC_MCF_HarmInject_uDcLnkBase_V
  Constant1 : Constant  Value=KfMDCC_MCF_HarmIn5_SpdLimHigh_rads
  Constant2 : Constant  Value=200  OutDataTypeStr=single
  Constant3 : Constant  Value=KfMDCC_MCF_HarmIn5_SpdLimLow_rads
  Constant4 : Constant  Value=100  OutDataTypeStr=single
  Constant5 : Constant  Value=200  OutDataTypeStr=single
  Constant6 : Constant  Value=KfMDCC_MCF_HarmIn5_SpdLimLow_rads
  Divide : Product  Inputs=*/*
  Logical Operator2 : Logic  AllPortsSameDT=off  OutDataTypeStr=boolean
  Logical Operator3 : Logic  Inputs=3  AllPortsSameDT=off  OutDataTypeStr=boolean
  Relational Operator : RelationalOperator  Operator=>  OutDataTypeStr=boolean  RndMeth=Simplest
  Relational Operator1 : RelationalOperator  Operator=<=  OutDataTypeStr=boolean  RndMeth=Simplest
  Relational Operator2 : RelationalOperator  Operator=<=  OutDataTypeStr=boolean  RndMeth=Simplest
  Relational Operator3 : RelationalOperator  Operator=>  OutDataTypeStr=boolean  RndMeth=Simplest
  Switch{4..8} (5 alike) : Switch  Criteria=u2 ~= 0
  Unit Delay2 : UnitDelay  SampleTime=-1  HasFrameUpgradeWarning=on
  Unit Delay3 : UnitDelay  SampleTime=-1  HasFrameUpgradeWarning=on
  Zero5 : Constant  Value=0  OutDataTypeStr=boolean
  Zero6 : Constant  OutDataTypeStr=boolean
  Zero7 : Constant  OutDataTypeStr=boolean
  Zero8 : Constant  Value=0  OutDataTypeStr=boolean
  Out2 : Outport
  wires:
  Constant/1 -> Divide/2
  MCF_uDcLnk/1 -> Divide/1
  Constant1/1 -> Switch4/3, Divide/3
  Divide/1 -> Switch4/1, Compare To Constant2/1
  Compare To Constant2/1 -> Switch4/2
  Switch4/1 -> [nLim]
  CAL_MCF_flgUse5Harm_b1/1 -> Logical Operator3/2
  Relational Operator2/1 -> Switch8/2
  Relational Operator1/1 -> Switch6/2
  Switch8/1 -> Switch7/3
  Compare To Constant7/1 -> Switch7/2
  Unit Delay3/1 -> Switch8/3
  Switch7/1 -> Unit Delay3/1, Logical Operator2/2
  Relational Operator/1 -> Switch5/2
  Switch5/1 -> Logical Operator2/1, Unit Delay2/1
  Zero6/1 -> Switch6/1
  Logical Operator3/1 -> Out2/1
  Switch6/1 -> Switch5/3
  Zero7/1 -> Switch7/1
  Unit Delay2/1 -> Switch6/3
  Zero8/1 -> Switch8/1
  Rdc_absnWoFlt_rads/1 -> Relational Operator/1, Relational Operator2/1, Compare To Constant7/1, Relational Operator1/1
  Logical Operator2/1 -> Logical Operator3/1
  Zero5/1 -> Switch5/1
  [nLim] -> Relational Operator/2
  [nLim] -> Add/1
  Add/1 -> Relational Operator1/2
  Constant2/1 -> Add/2
  Constant3/1 -> Add1/1
  Constant4/1 -> Add1/2
  Add1/1 -> Relational Operator2/2
  [nLim] -> Add2/1
  Constant5/1 -> Add2/2
  Add2/1 -> Relational Operator3/1
  Constant6/1 -> Relational Operator3/2
  Relational Operator3/1 -> Logical Operator3/3

== system MDCC/DoCurCtr_sys/MDCC/UdUqCalc_Sys/MDCC_MCF_Sys/Enabled Subsystem/Harmonic_Injection_5/Subsystem2 ==
  TDC_TrqDes : Inport
  flgHarmUse : Inport  Port=2
  Add : Sum  Inputs=+-
  Add1 : Sum  Inputs=-+
  Add2 : Sum  Inputs=-+
  Add3 : Sum
  Compare To Constant : simulink/Logic and Bit Operations/Compare To Constant  relop=>=  const=KfMDCC_MCF_TrqFltCof_NULL  OutDataTypeStr=boolean
  Compare To Constant1 : simulink/Logic and Bit Operations/Compare To Constant  relop=>=  const=KfMDCC_MCF_TrqFltCof_NULL  OutDataTypeStr=boolean
  Constant : Constant  Value=KfMDCC_MCF_TrqFlt_coef  OutDataTypeStr=single
  Switch : Switch  Criteria=u2 > Threshold
  Switch1 : Switch  Criteria=u2 > Threshold
  Switch2 : Switch  Criteria=u2 ~= 0
  Unit Delay : UnitDelay  SampleTime=-1  HasFrameUpgradeWarning=on
  Unit Delay1 : UnitDelay  SampleTime=-1  HasFrameUpgradeWarning=on
  Zero : Constant  Value=0  OutDataTypeStr=single
  TDC_TrqDesFlt : Outport
  wires:
  Add/1 -> Compare To Constant/1
  Compare To Constant/1 -> Switch/2
  Add1/1 -> Switch/1
  Switch/1 -> Switch2/1
  TDC_TrqDes/1 -> Switch1/3, Add2/2, Add/2
  Add2/1 -> Compare To Constant1/1
  Constant/1 -> Add3/1, Add1/1
  Add3/1 -> Switch1/1
  Compare To Constant1/1 -> Switch1/2
  Switch1/1 -> Switch/3
  Unit Delay/1 -> Add/1, Add1/2, Add2/1, Add3/2
  flgHarmUse/1 -> Unit Delay1/1
  Unit Delay1/1 -> Switch2/2
  Zero/1 -> Switch2/3
  Switch2/1 -> Unit Delay/1, TDC_TrqDesFlt/1

== system MDCC/DoCurCtr_sys/MDCC/UdUqCalc_Sys/MDCC_MCF_Sys/Enabled Subsystem/Harmonic_Injection_7/Set_7_steps_current_isdqdes ==
  TDC_TrqDesFlt : Inport
  1-D Lookup Table : Lookup_n-D  NumberOfTableDimensions=1  BreakpointsForDimension1=KfMDCC_MCF_HarmIn57ZRY_Trq_Nm  Table=KfMDCC_MCF_HarmIn7ZRY_Isd_A  InternalRulePriority=Speed  RndMeth=Simplest  InputSameDT=on
  1-D Lookup Table1 : Lookup_n-D  NumberOfTableDimensions=1  BreakpointsForDimension1=KfMDCC_MCF_HarmIn57ZRY_Trq_Nm  Table=KfMDCC_MCF_HarmIn7ZRY_Isq_A  InternalRulePriority=Speed  RndMeth=Simplest  InputSameDT=on
  Bus Creator1 : BusCreator  Inputs=2
  Bus Creator2 : BusCreator  Inputs=2
  Bus Selector1 : BusSelector  OutputSignals=MCF_IsdDes7Harm_A,MCF_IsqDes7Harm_A
  CAL_MCF_IsDes7Harm_f32 : Constant  Value=KfMDCC_MCF_IsDes7Harm_A
  CAL_MCF_IsThetaDes7Harm_f32 : Constant  Value=KfMDCC_MCF_IsThetaDes7Harm_NULL
  CAL_MCF_flgHarmInIsdqTab7ZR_b : Constant  Value=KbMDCC_MCF_flgHarmInIsdqTab7ZR_flg
  LookUpEAngleCosSin2 : Subsystem  TreatAsAtomicUnit=on  RTWFcnName=MCF_MDCC_LookUpEAngleCosSin  RTWFileName=MDCC
      settings: RTWFcnNameOpts=User specified
  Product2 : Product
  Product5 : Product
  Product7 : Product  OutDataTypeStr=uint16
  Signal Copy : SignalConversion  OverrideOpt=off
  Signal Copy1 : SignalConversion  OverrideOpt=off
  Sine_and_cosine_table1 : Constant  Value=7.357  OutDataTypeStr=single
  Switch1 : Switch  Criteria=u2 ~= 0
  VfMDCC_MCF_IsdDes7Harm_A : Outport  VectorParamsAs1DForOutWhenUnconnected=off
  VfMDCC_MCF_IsqDes7Harm_A : Outport  Port=2  VectorParamsAs1DForOutWhenUnconnected=off
  wires:
  Signal Copy1/1 -> VfMDCC_MCF_IsqDes7Harm_A/1  "VfMDCC_MCF_IsqDes7Harm_A"
  Signal Copy/1 -> VfMDCC_MCF_IsdDes7Harm_A/1  "VfMDCC_MCF_IsdDes7Harm_A"
  Bus Selector1/2 -> Signal Copy1/1  "<MCF_IsqDes7Harm_A>"
  Bus Selector1/1 -> Signal Copy/1  "<MCF_IsdDes7Harm_A>"
  Switch1/1 -> Bus Selector1/1
  CAL_MCF_flgHarmInIsdqTab7ZR_b/1 -> Switch1/2
  1-D Lookup Table1/1 -> Bus Creator2/2  "MCF_IsqDes7Harm_A"
  Bus Creator2/1 -> Switch1/1
  1-D Lookup Table/1 -> Bus Creator2/1  "MCF_IsdDes7Harm_A"
  TDC_TrqDesFlt/1 -> 1-D Lookup Table/1, 1-D Lookup Table1/1
  CAL_MCF_IsDes7Harm_f32/1 -> Product5/1, Product2/1
  Sine_and_cosine_table1/1 -> Product7/2
  LookUpEAngleCosSin2/2(VfMDCC_EAngleSin_NULL) -> Product5/2
  Product2/1 -> Bus Creator1/1  "MCF_IsdDes7Harm_A"
  Bus Creator1/1 -> Switch1/3
  Product7/1 -> LookUpEAngleCosSin2/1(VuMDCC_MotorPositionCnt_NULL)
  CAL_MCF_IsThetaDes7Harm_f32/1 -> Product7/1
  Product5/1 -> Bus Creator1/2  "MCF_IsqDes7Harm_A"
  LookUpEAngleCosSin2/1(VfMDCC_EAngleCos_NULL) -> Product2/2

== system MDCC/DoCurCtr_sys/MDCC/UdUqCalc_Sys/MDCC_MCF_Sys/Enabled Subsystem/Harmonic_Injection_7/Subsystem ==
  MCF_Harm_isdDes7 : Inport
  MCF_Harm_isqDes7 : Inport  Port=2
  MCF_Harm_isdAct7 : Inport  Port=3
  MCF_Harm_isqAct7 : Inport  Port=4
  MCF_Sin7Ag : Inport  Port=5
  MCF_Cos7Ag : Inport  Port=6
  Rdc_absnWoFlt_rads : Inport  Port=7
  MCF_flgHarm7PIRest : Inport  Port=8
  ZeroEnable : EnablePort
  Harm_7Step_KpKi : Subsystem
  RevPark : Subsystem
  MCF_uAlpha_Harm7 : Outport  VectorParamsAs1DForOutWhenUnconnected=off
  MCF_uBeta_Harm7 : Outport  Port=2  VectorParamsAs1DForOutWhenUnconnected=off
  wires:
  MCF_Harm_isqDes7/1 -> Harm_7Step_KpKi/2(MCF_Harm_isqDes7)
  MCF_Harm_isqAct7/1 -> Harm_7Step_KpKi/4(MCF_Harm_isqAct7)
  RevPark/2(MCF_uBeta_Harm7) -> MCF_uBeta_Harm7/1
  MCF_Harm_isdAct7/1 -> Harm_7Step_KpKi/3(MCF_Harm_isdAct7)
  RevPark/1(MCF_uAlpha_Harm7) -> MCF_uAlpha_Harm7/1
  MCF_Harm_isdDes7/1 -> Harm_7Step_KpKi/1(MCF_Harm_isdDes7)
  MCF_flgHarm7PIRest/1 -> Harm_7Step_KpKi/6(MCF_flgHarm7PIRest)
  Rdc_absnWoFlt_rads/1 -> Harm_7Step_KpKi/5(Rdc_absnWoFlt_rads)
  Harm_7Step_KpKi/1(MCF_Harm_ud7PI) -> RevPark/1(MCF_Harm_ud7PI)
  Harm_7Step_KpKi/2(MCF_Harm_uq7PI) -> RevPark/2(MCF_Harm_uq7PI)
  MCF_Sin7Ag/1 -> RevPark/3(MCF_Sin7Ag)
  MCF_Cos7Ag/1 -> RevPark/4(MCF_Cos7Ag)

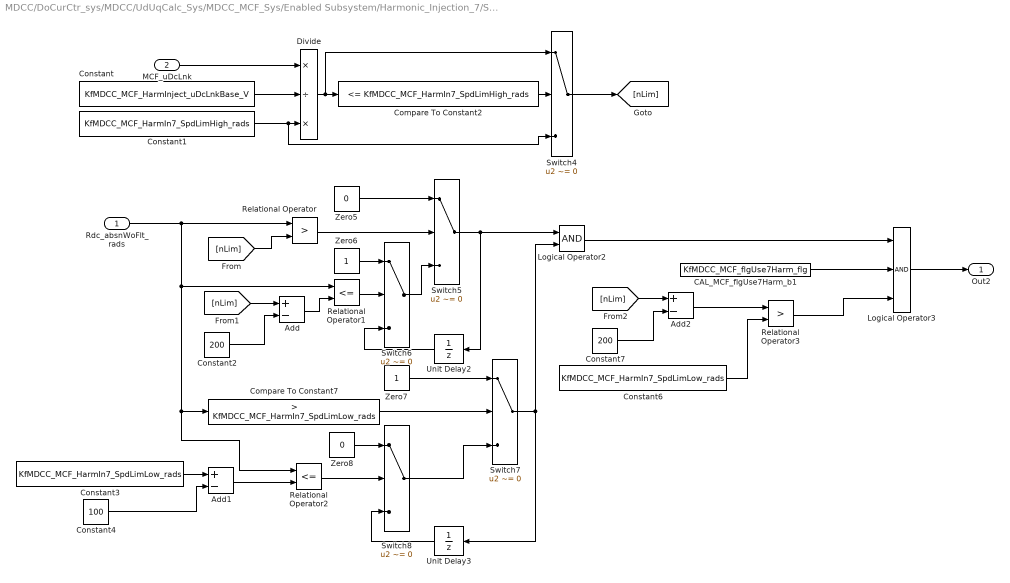
== system MDCC/DoCurCtr_sys/MDCC/UdUqCalc_Sys/MDCC_MCF_Sys/Enabled Subsystem/Harmonic_Injection_7/Subsystem1 ==
  Rdc_absnWoFlt_rads : Inport
  MCF_uDcLnk : Inport  Port=2
  Add : Sum  Inputs=+-
  Add1 : Sum  Inputs=+-
  Add2 : Sum  Inputs=+-
  CAL_MCF_flgUse7Harm_b1 : Constant  Value=KfMDCC_MCF_flgUse7Harm_flg
  Compare To Constant2 : simulink/Logic and Bit Operations/Compare To Constant  relop=<=  const=KfMDCC_MCF_HarmIn7_SpdLimHigh_rads  OutDataTypeStr=boolean
  Compare To Constant7 : simulink/Logic and Bit Operations/Compare To Constant  relop=>  const=KfMDCC_MCF_HarmIn7_SpdLimLow_rads  OutDataTypeStr=boolean
  Constant : Constant  Value=KfMDCC_MCF_HarmInject_uDcLnkBase_V
  Constant1 : Constant  Value=KfMDCC_MCF_HarmIn7_SpdLimHigh_rads
  Constant2 : Constant  Value=200  OutDataTypeStr=single
  Constant3 : Constant  Value=KfMDCC_MCF_HarmIn7_SpdLimLow_rads
  Constant4 : Constant  Value=100  OutDataTypeStr=single
  Constant6 : Constant  Value=KfMDCC_MCF_HarmIn7_SpdLimLow_rads
  Constant7 : Constant  Value=200  OutDataTypeStr=single
  Divide : Product  Inputs=*/*
  Logical Operator2 : Logic  AllPortsSameDT=off  OutDataTypeStr=boolean
  Logical Operator3 : Logic  Inputs=3  AllPortsSameDT=off  OutDataTypeStr=boolean
  Relational Operator : RelationalOperator  Operator=>  OutDataTypeStr=boolean  RndMeth=Simplest
  Relational Operator1 : RelationalOperator  Operator=<=  OutDataTypeStr=boolean  RndMeth=Simplest
  Relational Operator2 : RelationalOperator  Operator=<=  OutDataTypeStr=boolean  RndMeth=Simplest
  Relational Operator3 : RelationalOperator  Operator=>  OutDataTypeStr=boolean  RndMeth=Simplest
  Switch{4..8} (5 alike) : Switch  Criteria=u2 ~= 0
  Unit Delay2 : UnitDelay  SampleTime=-1  HasFrameUpgradeWarning=on
  Unit Delay3 : UnitDelay  SampleTime=-1  HasFrameUpgradeWarning=on
  Zero5 : Constant  Value=0  OutDataTypeStr=boolean
  Zero6 : Constant  OutDataTypeStr=boolean
  Zero7 : Constant  OutDataTypeStr=boolean
  Zero8 : Constant  Value=0  OutDataTypeStr=boolean
  Out2 : Outport
  wires:
  Constant/1 -> Divide/2
  MCF_uDcLnk/1 -> Divide/1
  Constant1/1 -> Switch4/3, Divide/3
  Divide/1 -> Switch4/1, Compare To Constant2/1
  Compare To Constant2/1 -> Switch4/2
  Switch4/1 -> [nLim]
  CAL_MCF_flgUse7Harm_b1/1 -> Logical Operator3/2
  Relational Operator2/1 -> Switch8/2
  Relational Operator1/1 -> Switch6/2
  Switch8/1 -> Switch7/3
  Compare To Constant7/1 -> Switch7/2
  Unit Delay3/1 -> Switch8/3
  Switch7/1 -> Unit Delay3/1, Logical Operator2/2
  Relational Operator/1 -> Switch5/2
  Switch5/1 -> Logical Operator2/1, Unit Delay2/1
  Zero6/1 -> Switch6/1
  Logical Operator3/1 -> Out2/1
  Switch6/1 -> Switch5/3
  Zero7/1 -> Switch7/1
  Unit Delay2/1 -> Switch6/3
  Zero8/1 -> Switch8/1
  Rdc_absnWoFlt_rads/1 -> Relational Operator/1, Relational Operator2/1, Compare To Constant7/1, Relational Operator1/1
  Logical Operator2/1 -> Logical Operator3/1
  Zero5/1 -> Switch5/1
  [nLim] -> Relational Operator/2
  [nLim] -> Add/1
  Add/1 -> Relational Operator1/2
  Constant2/1 -> Add/2
  Constant3/1 -> Add1/1
  Constant4/1 -> Add1/2
  Add1/1 -> Relational Operator2/2
  [nLim] -> Add2/1
  Constant7/1 -> Add2/2
  Add2/1 -> Relational Operator3/1
  Constant6/1 -> Relational Operator3/2
  Relational Operator3/1 -> Logical Operator3/3

== system MDCC/DoCurCtr_sys/MDCC/UdUqCalc_Sys/MDCC_MCF_Sys/Enabled Subsystem/Harmonic_Injection_7/Subsystem2 ==
  TDC_TrqDes : Inport
  flgHarmUse : Inport  Port=2
  Add : Sum  Inputs=+-
  Add1 : Sum  Inputs=-+
  Add2 : Sum  Inputs=-+
  Add3 : Sum
  Compare To Constant : simulink/Logic and Bit Operations/Compare To Constant  relop=>=  const=KfMDCC_MCF_TrqFltCof_NULL  OutDataTypeStr=boolean
  Compare To Constant1 : simulink/Logic and Bit Operations/Compare To Constant  relop=>=  const=KfMDCC_MCF_TrqFltCof_NULL  OutDataTypeStr=boolean
  Constant : Constant  Value=KfMDCC_MCF_TrqFlt_coef  OutDataTypeStr=single
  Switch : Switch  Criteria=u2 > Threshold
  Switch1 : Switch  Criteria=u2 > Threshold
  Switch2 : Switch  Criteria=u2 ~= 0
  Unit Delay : UnitDelay  SampleTime=-1  HasFrameUpgradeWarning=on
  Unit Delay1 : UnitDelay  SampleTime=-1  HasFrameUpgradeWarning=on
  Zero : Constant  Value=0  OutDataTypeStr=single
  TDC_TrqDesFlt : Outport
  wires:
  Add/1 -> Compare To Constant/1
  Compare To Constant/1 -> Switch/2
  Add1/1 -> Switch/1
  Switch/1 -> Switch2/1
  TDC_TrqDes/1 -> Switch1/3, Add2/2, Add/2
  Add2/1 -> Compare To Constant1/1
  Constant/1 -> Add1/1, Add3/1
  Add3/1 -> Switch1/1
  Compare To Constant1/1 -> Switch1/2
  Switch1/1 -> Switch/3
  Unit Delay/1 -> Add/1, Add1/2, Add2/1, Add3/2
  flgHarmUse/1 -> Unit Delay1/1
  Unit Delay1/1 -> Switch2/2
  Zero/1 -> Switch2/3
  Switch2/1 -> Unit Delay/1, TDC_TrqDesFlt/1

== system MDCC/DoCurCtr_sys/MDCC/UdUqCalc_Sys/MDCC_MCF_Sys/Enabled Subsystem/Subsystem1/Park11 ==
  note: 低通滤波器
  MCF_AgSin : Inport
  MCF_ialpha_Harm : Inport  Port=2
  MCF_ibeta_Harm : Inport  Port=3
  MCF_AgCos : Inport  Port=4
  MCF_dtPWM : Inport  Port=5
  dB_Harm : Inport  Port=6
  Add : Sum
  Add1 : Sum  Inputs=-+
  Product{,1..3} (4 alike) : Product
  Subsystem : Subsystem
  Subsystem1 : Subsystem
  MCF_Id_Harm : Outport
  MCF_Iq_Harm : Outport  Port=2
  wires:
  Add/1 -> Subsystem/1(In1)
  Add1/1 -> Subsystem1/3(In1)
  Product2/1 -> Add1/1
  Product/1 -> Add/1
  Product1/1 -> Add/2
  Product3/1 -> Add1/2
  Subsystem/1(Out1) -> MCF_Id_Harm/1
  Subsystem1/1(Out1) -> MCF_Iq_Harm/1
  MCF_ialpha_Harm/1 -> Product2/1, Product/1
  MCF_AgCos/1 -> Product/2, Product3/2
  MCF_ibeta_Harm/1 -> Product1/1, Product3/1
  MCF_AgSin/1 -> Product1/2, Product2/2
  MCF_dtPWM/1 -> Subsystem1/2(MCF_dtPWM), Subsystem/2(MCF_dtPWM)
  dB_Harm/1 -> Subsystem/3(dB_Harm), Subsystem1/1(dB_Harm)

== system MDCC/DoCurCtr_sys/MDCC/UdUqCalc_Sys/MDCC_MCF_Sys/Enabled Subsystem/Subsystem1/Park13 ==
  note: 低通滤波器
  MCF_AgSin : Inport
  MCF_ialpha_Harm : Inport  Port=2
  MCF_ibeta_Harm : Inport  Port=3
  MCF_AgCos : Inport  Port=4
  MCF_dtPWM : Inport  Port=5
  dB_Harm : Inport  Port=6
  Add : Sum
  Add1 : Sum  Inputs=-+
  Product{,1..3} (4 alike) : Product
  Subsystem : Subsystem
  Subsystem1 : Subsystem
  MCF_Id_Harm : Outport
  MCF_Iq_Harm : Outport  Port=2
  wires:
  Add/1 -> Subsystem/1(In1)
  Add1/1 -> Subsystem1/3(In1)
  Product2/1 -> Add1/1
  Product/1 -> Add/1
  Product1/1 -> Add/2
  Product3/1 -> Add1/2
  Subsystem/1(Out1) -> MCF_Id_Harm/1
  Subsystem1/1(Out1) -> MCF_Iq_Harm/1
  MCF_ialpha_Harm/1 -> Product2/1, Product/1
  MCF_AgCos/1 -> Product/2, Product3/2
  MCF_ibeta_Harm/1 -> Product1/1, Product3/1
  MCF_AgSin/1 -> Product1/2, Product2/2
  MCF_dtPWM/1 -> Subsystem1/2(MCF_dtPWM), Subsystem/2(MCF_dtPWM)
  dB_Harm/1 -> Subsystem/3(dB_Harm), Subsystem1/1(dB_Harm)

== system MDCC/DoCurCtr_sys/MDCC/UdUqCalc_Sys/MDCC_MCF_Sys/Enabled Subsystem/Subsystem1/Park5 ==
  note: 低通滤波器
  MCF_AgSin : Inport
  MCF_ialpha_Harm : Inport  Port=2
  MCF_ibeta_Harm : Inport  Port=3
  MCF_AgCos : Inport  Port=4
  MCF_dtPWM : Inport  Port=5
  dB_Harm : Inport  Port=6
  Add : Sum
  Add1 : Sum  Inputs=-+
  Product{,1..3} (4 alike) : Product
  Subsystem : Subsystem
  Subsystem1 : Subsystem
  MCF_Id_Harm : Outport
  MCF_Iq_Harm : Outport  Port=2
  wires:
  Add/1 -> Subsystem/1(In1)
  Add1/1 -> Subsystem1/3(In1)
  Product2/1 -> Add1/1
  Product/1 -> Add/1
  Product1/1 -> Add/2
  Product3/1 -> Add1/2
  Subsystem/1(Out1) -> MCF_Id_Harm/1
  Subsystem1/1(Out1) -> MCF_Iq_Harm/1
  MCF_ialpha_Harm/1 -> Product2/1, Product/1
  MCF_AgCos/1 -> Product/2, Product3/2
  MCF_ibeta_Harm/1 -> Product1/1, Product3/1
  MCF_AgSin/1 -> Product1/2, Product2/2
  MCF_dtPWM/1 -> Subsystem1/2(MCF_dtPWM), Subsystem/2(MCF_dtPWM)
  dB_Harm/1 -> Subsystem/3(dB_Harm), Subsystem1/1(dB_Harm)

== system MDCC/DoCurCtr_sys/MDCC/UdUqCalc_Sys/MDCC_MCF_Sys/Enabled Subsystem/Subsystem1/Park7 ==
  note: 低通滤波器
  MCF_AgSin : Inport
  MCF_ialpha_Harm : Inport  Port=2
  MCF_ibeta_Harm : Inport  Port=3
  MCF_AgCos : Inport  Port=4
  MCF_dtPWM : Inport  Port=5
  dB_Harm : Inport  Port=6
  Add : Sum
  Add1 : Sum  Inputs=-+
  Product{,1..3} (4 alike) : Product
  Subsystem : Subsystem
  Subsystem1 : Subsystem
  MCF_Id_Harm : Outport
  MCF_Iq_Harm : Outport  Port=2
  wires:
  Add/1 -> Subsystem/1(In1)
  Add1/1 -> Subsystem1/3(In1)
  Product2/1 -> Add1/1
  Product/1 -> Add/1
  Product1/1 -> Add/2
  Product3/1 -> Add1/2
  Subsystem/1(Out1) -> MCF_Id_Harm/1
  Subsystem1/1(Out1) -> MCF_Iq_Harm/1
  MCF_ialpha_Harm/1 -> Product2/1, Product/1
  MCF_AgCos/1 -> Product/2, Product3/2
  MCF_ibeta_Harm/1 -> Product1/1, Product3/1
  MCF_AgSin/1 -> Product1/2, Product2/2
  MCF_dtPWM/1 -> Subsystem1/2(MCF_dtPWM), Subsystem/2(MCF_dtPWM)
  dB_Harm/1 -> Subsystem/3(dB_Harm), Subsystem1/1(dB_Harm)

== system MDCC/DoCurCtr_sys/MDCC/UdUqCalc_Sys/MDCC_MCF_Sys/Enabled Subsystem/Subsystem1/Subsystem ==
  VuMDCC_MotorPositionCnt_NULL : Inport
  Coeficientof11axis : Constant  Value=-11  OutDataTypeStr=single
  Coeficientof13axis : Constant  Value=13  OutDataTypeStr=single
  Coeficientof5axis : Constant  Value=-5  OutDataTypeStr=single
  Coeficientof7axis : Constant  Value=7  OutDataTypeStr=single
  Constant{,1..3} (4 alike) : Constant  Value=4095  OutDataTypeStr=single
  Data Type Conversion : DataTypeConversion  OutDataTypeStr=single
  Data Type Conversion{1..4} (4 alike) : DataTypeConversion  OutDataTypeStr=uint16
  LookUpEAngleCosSin1 : Subsystem  TreatAsAtomicUnit=on  RTWFcnName=MCF_MDCC_LookUpEAngleCosSin  RTWFileName=MDCC
      settings: RTWFcnNameOpts=User specified
  LookUpEAngleCosSin2 : Subsystem  TreatAsAtomicUnit=on  RTWFcnName=MCF_MDCC_LookUpEAngleCosSin  RTWFileName=MDCC
      settings: RTWFcnNameOpts=User specified
  LookUpEAngleCosSin3 : Subsystem  TreatAsAtomicUnit=on  RTWFcnName=MCF_MDCC_LookUpEAngleCosSin  RTWFileName=MDCC
      settings: RTWFcnNameOpts=User specified
  LookUpEAngleCosSin5 : Subsystem  TreatAsAtomicUnit=on  RTWFcnName=MCF_MDCC_LookUpEAngleCosSin  RTWFileName=MDCC
      settings: RTWFcnNameOpts=User specified
  Mod{,1..3} (4 alike) : Math  Operator=mod  SaturateOnIntegerOverflow=on
  Product{3..6} (4 alike) : Product
  MCF_AgSin5 : Outport
  MCF_AgCos5 : Outport  Port=2
  MCF_AgSin7 : Outport  Port=3
  MCF_AgCos7 : Outport  Port=4
  MCF_AgSin11 : Outport  Port=5
  MCF_AgCos11 : Outport  Port=6
  MCF_AgSin13 : Outport  Port=7
  MCF_AgCos13 : Outport  Port=8
  wires:
  Coeficientof5axis/1 -> Product3/2
  LookUpEAngleCosSin2/1(VfMDCC_EAngleCos_NULL) -> MCF_AgSin5/1
  LookUpEAngleCosSin2/2(VfMDCC_EAngleSin_NULL) -> MCF_AgCos5/1
  Coeficientof7axis/1 -> Product4/2
  LookUpEAngleCosSin5/2(VfMDCC_EAngleSin_NULL) -> MCF_AgCos7/1
  LookUpEAngleCosSin5/1(VfMDCC_EAngleCos_NULL) -> MCF_AgSin7/1
  Coeficientof11axis/1 -> Product5/2
  LookUpEAngleCosSin1/2(VfMDCC_EAngleSin_NULL) -> MCF_AgCos11/1
  LookUpEAngleCosSin1/1(VfMDCC_EAngleCos_NULL) -> MCF_AgSin11/1
  Coeficientof13axis/1 -> Product6/2
  VuMDCC_MotorPositionCnt_NULL/1 -> Data Type Conversion/1
  LookUpEAngleCosSin3/1(VfMDCC_EAngleCos_NULL) -> MCF_AgSin13/1
  LookUpEAngleCosSin3/2(VfMDCC_EAngleSin_NULL) -> MCF_AgCos13/1
  Data Type Conversion/1 -> Product6/1, Product5/1, Product4/1, Product3/1
  Constant/1 -> Mod/2
  Constant1/1 -> Mod1/2
  Constant2/1 -> Mod2/2
  Constant3/1 -> Mod3/2
  Product4/1 -> Mod1/1
  Product6/1 -> Mod3/1
  Product5/1 -> Mod2/1
  Product3/1 -> Mod/1
  Mod1/1 -> Data Type Conversion2/1
  Mod/1 -> Data Type Conversion4/1
  Mod2/1 -> Data Type Conversion3/1
  Mod3/1 -> Data Type Conversion1/1
  Data Type Conversion1/1 -> LookUpEAngleCosSin3/1(VuMDCC_MotorPositionCnt_NULL)
  Data Type Conversion3/1 -> LookUpEAngleCosSin1/1(VuMDCC_MotorPositionCnt_NULL)
  Data Type Conversion2/1 -> LookUpEAngleCosSin5/1(VuMDCC_MotorPositionCnt_NULL)
  Data Type Conversion4/1 -> LookUpEAngleCosSin2/1(VuMDCC_MotorPositionCnt_NULL)

== system MDCC/DoCurCtr_sys/MDCC/UdUqCalc_Sys/MDCC_MCF_Sys/Enabled Subsystem/Subsystem2/Mcf_AgTranCalc11 ==
  Harm_AgCpn : Inport
  Harm_coef : Inport  Port=2
  Constant : Constant  Value=4095  OutDataTypeStr=single
  Data Type Conversion : DataTypeConversion  OutDataTypeStr=uint16
  Divide2 : Product  Inputs=**  OutDataTypeStr=single
  LookUpEAngleCosSin2 : Subsystem  TreatAsAtomicUnit=on  RTWFcnName=MCF_MDCC_LookUpEAngleCosSin  RTWFileName=MDCC
      settings: RTWFcnNameOpts=User specified
  Mod : Math  Operator=mod  SaturateOnIntegerOverflow=on
  MCF_SinAg : Outport  VectorParamsAs1DForOutWhenUnconnected=off
  MCF_CosAg : Outport  Port=2  VectorParamsAs1DForOutWhenUnconnected=off
  wires:
  LookUpEAngleCosSin2/2(VfMDCC_EAngleSin_NULL) -> MCF_CosAg/1  "MCF_CosAg"
  LookUpEAngleCosSin2/1(VfMDCC_EAngleCos_NULL) -> MCF_SinAg/1  "MCF_SinAg"
  Harm_AgCpn/1 -> Divide2/1
  Divide2/1 -> Mod/1
  Constant/1 -> Mod/2
  Harm_coef/1 -> Divide2/2
  Mod/1 -> Data Type Conversion/1
  Data Type Conversion/1 -> LookUpEAngleCosSin2/1(VuMDCC_MotorPositionCnt_NULL)

== system MDCC/DoCurCtr_sys/MDCC/UdUqCalc_Sys/MDCC_MCF_Sys/Enabled Subsystem/Subsystem2/Mcf_AgTranCalc13 ==
  Harm_AgCpn : Inport
  Harm_coef : Inport  Port=2
  Constant : Constant  Value=4095  OutDataTypeStr=single
  Data Type Conversion : DataTypeConversion  OutDataTypeStr=uint16
  Divide2 : Product  Inputs=**  OutDataTypeStr=single
  LookUpEAngleCosSin2 : Subsystem  TreatAsAtomicUnit=on  RTWFcnName=MCF_MDCC_LookUpEAngleCosSin  RTWFileName=MDCC
      settings: RTWFcnNameOpts=User specified
  Mod : Math  Operator=mod  SaturateOnIntegerOverflow=on
  MCF_SinAg : Outport  VectorParamsAs1DForOutWhenUnconnected=off
  MCF_CosAg : Outport  Port=2  VectorParamsAs1DForOutWhenUnconnected=off
  wires:
  LookUpEAngleCosSin2/2(VfMDCC_EAngleSin_NULL) -> MCF_CosAg/1  "MCF_CosAg"
  LookUpEAngleCosSin2/1(VfMDCC_EAngleCos_NULL) -> MCF_SinAg/1  "MCF_SinAg"
  Harm_AgCpn/1 -> Divide2/1
  Divide2/1 -> Mod/1
  Constant/1 -> Mod/2
  Harm_coef/1 -> Divide2/2
  Mod/1 -> Data Type Conversion/1
  Data Type Conversion/1 -> LookUpEAngleCosSin2/1(VuMDCC_MotorPositionCnt_NULL)

== system MDCC/DoCurCtr_sys/MDCC/UdUqCalc_Sys/MDCC_MCF_Sys/Enabled Subsystem/Subsystem2/Mcf_AgTranCalc5 ==
  Harm_AgCpn : Inport
  Harm_coef : Inport  Port=2
  Constant : Constant  Value=4095  OutDataTypeStr=single
  Data Type Conversion : DataTypeConversion  OutDataTypeStr=uint16
  Divide2 : Product  Inputs=**  OutDataTypeStr=single
  LookUpEAngleCosSin2 : Subsystem  TreatAsAtomicUnit=on  RTWFcnName=MCF_MDCC_LookUpEAngleCosSin  RTWFileName=MDCC
      settings: RTWFcnNameOpts=User specified
  Mod : Math  Operator=mod  SaturateOnIntegerOverflow=on
  MCF_SinAg : Outport  VectorParamsAs1DForOutWhenUnconnected=off
  MCF_CosAg : Outport  Port=2  VectorParamsAs1DForOutWhenUnconnected=off
  wires:
  LookUpEAngleCosSin2/2(VfMDCC_EAngleSin_NULL) -> MCF_CosAg/1  "MCF_CosAg"
  LookUpEAngleCosSin2/1(VfMDCC_EAngleCos_NULL) -> MCF_SinAg/1  "MCF_SinAg"
  Harm_AgCpn/1 -> Divide2/1
  Divide2/1 -> Mod/1
  Constant/1 -> Mod/2
  Harm_coef/1 -> Divide2/2
  Mod/1 -> Data Type Conversion/1
  Data Type Conversion/1 -> LookUpEAngleCosSin2/1(VuMDCC_MotorPositionCnt_NULL)

== system MDCC/DoCurCtr_sys/MDCC/UdUqCalc_Sys/MDCC_MCF_Sys/Enabled Subsystem/Subsystem2/Mcf_AgTranCalc7 ==
  Harm_AgCpn : Inport
  Harm_coef : Inport  Port=2
  Constant : Constant  Value=4095  OutDataTypeStr=single
  Data Type Conversion : DataTypeConversion  OutDataTypeStr=uint16
  Divide2 : Product  Inputs=**  OutDataTypeStr=single
  LookUpEAngleCosSin2 : Subsystem  TreatAsAtomicUnit=on  RTWFcnName=MCF_MDCC_LookUpEAngleCosSin  RTWFileName=MDCC
      settings: RTWFcnNameOpts=User specified
  Mod : Math  Operator=mod  SaturateOnIntegerOverflow=on
  MCF_SinAg : Outport  VectorParamsAs1DForOutWhenUnconnected=off
  MCF_CosAg : Outport  Port=2  VectorParamsAs1DForOutWhenUnconnected=off
  wires:
  LookUpEAngleCosSin2/2(VfMDCC_EAngleSin_NULL) -> MCF_CosAg/1  "MCF_CosAg"
  LookUpEAngleCosSin2/1(VfMDCC_EAngleCos_NULL) -> MCF_SinAg/1  "MCF_SinAg"
  Harm_AgCpn/1 -> Divide2/1
  Divide2/1 -> Mod/1
  Constant/1 -> Mod/2
  Harm_coef/1 -> Divide2/2
  Mod/1 -> Data Type Conversion/1
  Data Type Conversion/1 -> LookUpEAngleCosSin2/1(VuMDCC_MotorPositionCnt_NULL)

== system MDCC/DoCurCtr_sys/MDCC/UdUqCalc_Sys/MDCC_MCF_Sys/Enabled Subsystem/Subsystem2/Subsystem ==
  HSPF_nSlowFlt : Inport
  dtPwmWoRpwm : Inport  Port=2
  MCF_agRtrEe : Inport  Port=3
  Add : Sum
  CAL_MCF_Harm_CpnAg_f32 : Constant  Value=KfMDCC_MCF_HarmCpnAg_NULL
  Constant : Constant  Value=4095  OutDataTypeStr=single
  Data Type Conversion : DataTypeConversion  OutDataTypeStr=single
  Divide1 : Product  Inputs=*/  OutDataTypeStr=Inherit: Same as first input
  First_LowPass : Subsystem
  Gain : Gain  Gain=pi/2048  OutDataTypeStr=single
  MCF_GLB_CircAge_f32 : Constant  Value=KfMDCC_MCF_CircAge_NULL
  MCF_GLB_Sixty_f3 : Constant  Value=2*pi  OutDataTypeStr=single
  Mod : Math  Operator=mod  SaturateOnIntegerOverflow=on
  Product : Product  OutDataTypeStr=single
  Product1 : Product
  Product2 : Product
  Harm_AgCpn : Outport
  wires:
  CAL_MCF_Harm_CpnAg_f32/1 -> Product/1
  HSPF_nSlowFlt/1 -> First_LowPass/1(MCF_n)
  Divide1/1 -> Product2/1  "MCF_frqStr"
  First_LowPass/1(MCF_nFlt) -> Divide1/1
  MCF_GLB_Sixty_f3/1 -> Divide1/2
  Product/1 -> Product2/2
  MCF_GLB_CircAge_f32/1 -> Product1/2
  Product2/1 -> Product1/1
  dtPwmWoRpwm/1 -> Product/2
  Product1/1 -> Gain/1
  Add/1 -> Mod/1
  MCF_agRtrEe/1 -> Data Type Conversion/1
  Gain/1 -> Add/1
  Mod/1 -> Harm_AgCpn/1
  Constant/1 -> Mod/2
  Data Type Conversion/1 -> Add/2

== system MDCC/DoCurCtr_sys/MDCC/UdUqCalc_Sys/SelfHeating/Subsystem1/Subsystem1/Subsystem1 ==
  set : Inport
  rate : Inport  Port=2
  this_ref : Inport  Port=3
  Add : Sum  OutDataTypeStr=single
  Data Type Conversion : DataTypeConversion  OutDataTypeStr=single
  MinMax : MinMax  Inputs=2  OutDataTypeStr=single
  MinMax1 : MinMax  Function=max  Inputs=2
  Subtract : Sum  Inputs=+-
  VfMDTM_SelfHeatingUdVal_V : Outport
  wires:
  rate/1 -> Subtract/2, Add/2
  MinMax1/1 -> VfMDTM_SelfHeatingUdVal_V/1
  this_ref/1 -> Subtract/1, Add/1
  set/1 -> Data Type Conversion/1
  Add/1 -> MinMax/2
  Subtract/1 -> MinMax1/2
  MinMax/1 -> MinMax1/1
  Data Type Conversion/1 -> MinMax/1
